simulink model "Gas_Turbine_Model_2017a_non_linear_PID"  (R2021a)
settings: Solver=ode15s  StartTime=0.0  StopTime=90000  FixedStep=0.001  RelTol=1e-3  EnableMultiTasking=on
values from neighbouring files (symbols this model uses):
  Beta_cmp = [1 1.5 2 2.5 3 3.5 4 4.5 5 5.5 6 6.5 ... (39 elements, 39x1)]    [Compressor_Map.mat]
  Eps_turb = [1 1.1 1.2 1.3 1.4 1.5 1.6 1.7 1.8 1.9 2 2.1 ... (191 elements, 1x191)]    [Turbine_Map.mat]
  Eta_cmp = [0.3 0.3 0.3 0.3 0.3 0.3 0.3 0.3 0.3 0.3 0.3 0.3 ... (585 elements, 15x39)]    [Compressor_Map.mat]
  Eta_turb = [0.586812592498 0.603057586725 0.61630240991 0.627098016156 0.635894182286 0.643058088048 0.648889484257 0.653633075447 0.657488628582 0.660619225395 0.663157999268 0.665213634952 ... (191 elements, 1x191)]    [Turbine_Map.mat]
  Mf_cmp = [0.246355651063 0.246355651063 0.246355651063 0.545009157509 1.57043960559 2.28211167924 2.75423550256 3.06528661824 3.27199659823 3.41123925415 3.50631480113 3.5719685441 ... (585 elements, 15x39)]    [Compressor_Map.mat]
  Mf_turb = [1.2124442703 1.39720469175 1.56286841441 1.71140925877 1.84459703271 1.96401861808 2.07109687783 2.16710760884 2.25319474261 2.3303839747 2.39959498557 2.4616523982 ... (191 elements, 1x191)]    [Turbine_Map.mat]
  N_cmp = [30000 35000 40000 45000 50000 55000 60000 65000 70000 75000 80000 85000 ... (15 elements, 1x15)]    [Compressor_Map.mat]
  pow_data = [49.5930192012 49.5930192012 47.1446947685 44.6063090759 42.0564349089 41.1061528351 40.7107031585 40.3152534819 41.8635649412 43.5549903366 45.246415732 45.7100796532 ... (145 elements, 1x145)]    [Pow_demand.mat]
  time_data = [0 600 1200 1800 2400 3000 3600 4200 4800 5400 6000 6600 ... (145 elements, 1x145)]    [Pow_demand.mat]
undefined symbols (not defined in the file or in its folder): cp, cp_m, cv, J, lambda, mf, pamb, Q_LHV, R, sigbuilder_block, Tamb, V
libraries: pid_lib x1
settings Model: Creator=Xinmin Zhang  LastModifiedBy=sandeepsulake
settings SolverCC: ZeroCrossAlgorithm=Adaptive  AlgebraicLoopSolver=TrustRegion
settings DataIOCC: LimitDataPoints=on  SaveFormat=Array  SignalLoggingSaveFormat=ModelDataLogs  ReturnWorkspaceOutputs=off
settings OptimizationCC: ExpressionDepthLimit=2147483647  LifeSpan=inf
settings DebuggingCC: AlgebraicLoopMsg=error  UnderspecifiedInitializationDetection=Classic  MergeDetectMultiDrivingBlocksExec=none  FcnCallInpInsideContextMsg=warning  StateNameClashWarn=warning  SFUnexpectedBacktrackingDiag=warning  SFNoUnconditionalDefaultTransitionDiag=warning  SFExecutionAtInitializationDiag=none  SFMachineParentedDataDiag=warning  ArithmeticOperatorsInVariantConditions=warning
settings HardwareCC: ProdBitPerPointer=32  ProdBitPerSizeT=32  ProdBitPerPtrDiffT=32  ProdLargestAtomicFloat=None  ProdIntDivRoundTo=Undefined  ProdEndianess=Unspecified  ProdWordSize=32  ProdHWDeviceType=32-bit Generic
settings ModelReferenceCC: PropagateSignalLabelsOutOfModel=off
settings SFSimCC: SimUseLocalCustomCode=off  CustomCodeUndefinedFunction=UseInterfaceOnly
settings RTWCC: RTWUseLocalCustomCode=off
settings CodeAppCC: StateflowObjectComments=on
settings GRTTargetCC: TargetLangStandard=C89/C90 (ANSI)  CombineOutputUpdateFcns=off  GRTInterface=on
settings ConfigComp: CovMetricSettings=dw  CovSaveCumulativeToWorkspaceVar=on  CovSaveSingleToWorkspaceVar=on  CovExternalEMLEnable=off

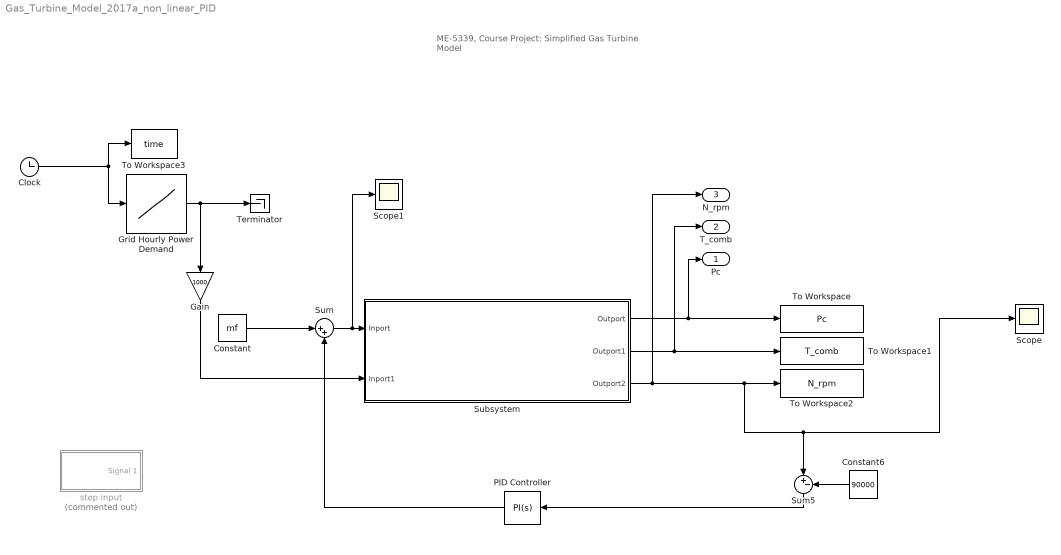
== system Gas_Turbine_Model_2017a_non_linear_PID ==
  note: ME-5339, Course Project:
      | Simplified Gas Turbine Model
  Clock : Clock
  Constant : Constant  Value=mf
  Constant6 : Constant  Value=90000
  Gain : Gain  Gain=1000
  Grid Hourly Power Demand : Lookup_n-D  NumberOfTableDimensions=1  BreakpointsForDimension1=time_data  Table=pow_data  RndMeth=Simplest  InputSameDT=on
  PID Controller : pid_lib/PID Controller  Controller=PI  Form=Parallel  TimeDomain=Continuous-time  UseExternalTs=off  SampleTime=-1  IntegratorMethod=Forward Euler  FilterMethod=Forward Euler  ControllerParametersSource=internal  P=-6.19982666191308e-06  I=-7.95045258926056e-07  D=0  UseFilter=on  N=100  TunerSelectOption=Transfer Function Based (PID Tuner App)  InitialConditionSource=internal  InitialConditionForIntegrator=0  InitialConditionForFilter=0  DifferentiatorICPrevScaledInput=0  ExternalReset=none  TrackingMode=off  Kt=1  LimitOutput=off  SatLimitsSource=internal  UpperSaturationLimit=inf  LowerSaturationLimit=0  LinearizeAsGain=on  AntiWindupMode=none  Kb=1  POutMin=[]  POutMax=[]  IOutMin=[]  IOutMax=[]  DOutMin=[]  DOutMax=[]  NOutMin=[]  NOutMax=[]  SumOutMin=[]  SumOutMax=[]  SaturationOutMin=[]  SaturationOutMax=[]  PParamMin=[]  PParamMax=[]  IParamMin=[]  IParamMax=[]  DParamMin=[]  DParamMax=[]  NParamMin=[]  NParamMax=[]  KbParamMin=[]  KbParamMax=[]  KtParamMin=[]  KtParamMax=[]  KbOutMin=[]  KbOutMax=[]  KtOutMin=[]  KtOutMax=[]  IntegratorOutMin=[]  IntegratorOutMax=[]  FilterOutMin=[]  FilterOutMax=[]  SumI1OutMin=[]  SumI1OutMax=[]  SumI2OutMin=[]  SumI2OutMax=[]  SumI3OutMin=[]  SumI3OutMax=[]  SumI4OutMin=[]  SumI4OutMax=[]  SumDOutMin=[]  SumDOutMax=[]  DifferentiatorOutMin=[]  DifferentiatorOutMax=[]  FilterDiffOutCoefMin=[]  FilterDiffOutCoefMax=[]  ReciprocalOutMin=[]  ReciprocalOutMax=[]  SumDenOutMin=[]  SumDenOutMax=[]  SumNumOutMin=[]  SumNumOutMax=[]  DivideOutMin=[]  DivideOutMax=[]  UdiffTsProdOutMin=[]  UdiffTsProdOutMax=[]  NTsProdOutMin=[]  NTsProdOutMax=[]  UintegralTsProdOutMin=[]  UintegralTsProdOutMax=[]  UngainTsProdOutMin=[]  UngainTsProdOutMax=[]  IntegratorContinuousStateAttributes=''  IntegratorStateMustResolveToSignalObject=off  IntegratorRTWStateStorageClass=Auto  FilterContinuousStateAttributes=''  FilterStateMustResolveToSignalObject=off  FilterRTWStateStorageClass=Auto  ParallelPVariant=InternalParameters  IdealPVariant=Disabled  IVariant=InternalParameters  DVariant=Disabled  IntegratorVariant=Continuous  SatVariant=Disabled  AWVariant=Passthrough  PCopyVariant=Disabled  TRVariant=Disabled  FdbkBlocksVariant=Forward  IdealPFdbkVariant=Disabled  SatFdbkVariant=Disabled  DerivativeFilterVariant=Disabled  NVariant=Disabled  NCopyVariant=Disabled_SignalSpec  FilterICVariant=Disabled  IntegratorICVariant=InternalICs  ExternalResetVariant=Disabled  TRSumVariant=Passthrough  SumFdbkVariant=Disabled  SumVariant=Sum_PI  TsampFilterVariant=InternalTs  TsampNgainVariant=Passthrough  TsampIntegralVariant=Passthrough  ExternalSaturationOutDataTypeStr=Inherit: Same as second input
  Scope : Scope
  Scope1 : Scope
  Subsystem : Subsystem
  Sum : Sum  Inputs=|++
  Sum5 : Sum  Inputs=|+-
  Terminator : Terminator
  To Workspace : ToWorkspace  VariableName=Pc  SampleTime=-1
  To Workspace1 : ToWorkspace  VariableName=T_comb  SampleTime=-1
  To Workspace2 : ToWorkspace  VariableName=N_rpm  SampleTime=-1
  To Workspace3 : ToWorkspace  VariableName=time  SampleTime=-1
  step input : Subsystem  Tag=STV Subsys  Commented=on  LoadFcn=sigbuilder_block('load');  StartFcn=sigbuilder_block('start');  StopFcn=sigbuilder_block('stop');  ClipboardFcn=sigbuilder_block('clipboard');  mask(Sigbuilder block){tuvar=[0:10]}
      mask help: Simulink:masks:SigbuilderBlock_MD
      mask init:
      | if ~strcmp(get_param(bdroot(gcbh),'SimulationStatus'),'stopped') tuvar = sigbuilder_block('maskInit'); end
      settings: CopyFcn=sigbuilder_block('copy');  DeleteFcn=sigbuilder_block('delete');  ModelCloseFcn=sigbuilder_block('modelClose');  PreSaveFcn=sigbuilder_block('preSave');  PauseFcn=sigbuilder_block('pause');  ContinueFcn=sigbuilder_block('continue');  NameChangeFcn=sigbuilder_block('namechange');  OpenFcn=sigbuilder_block('open',[437.6 199.2 550.4 400 ]);  CloseFcn=sigbuilder_block('close');
      mask Display: plot(0, 0, 100, 100,[2, 2, 32, 32, 2], [68, 8, 8, 68, 68],[32, 2], [38, 38], [32, 19, 2],[53, 60, 44], [32, 17, 17, 2],[16, 16, 31, 31]);txt = getActiveGroup(gcbh);text(2, 100, txt,'verticalAlignment', 'top');
  Pc : Outport
  T_comb : Outport  Port=2
  N_rpm : Outport  Port=3
  wires:
  Clock/1 -> To Workspace3/1, Grid Hourly Power Demand/1
  Grid Hourly Power Demand/1 -> Terminator/1, Gain/1
  Subsystem/1(Outport) -> Pc/1, To Workspace/1
  Subsystem/2(Outport1) -> T_comb/1, To Workspace1/1
  Constant/1 -> Sum/1
  Sum5/1 -> PID Controller/1
  Constant6/1 -> Sum5/2
  Subsystem/3(Outport2) -> Scope/1, Sum5/1, To Workspace2/1, N_rpm/1
  PID Controller/1 -> Sum/2
  Sum/1 -> Scope1/1, Subsystem/1(Inport)
  Gain/1 -> Subsystem/2(Inport1)

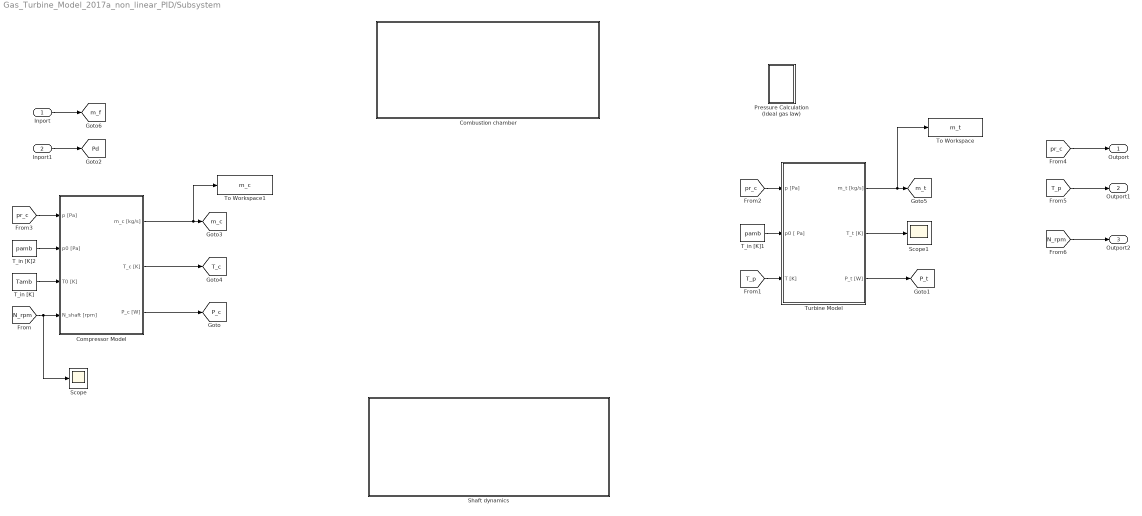
== system Gas_Turbine_Model_2017a_non_linear_PID/Subsystem ==
  Inport : Inport
  Inport1 : Inport  Port=2
  Combustion chamber : Subsystem
  Compressor Model : Subsystem
      mask help: Model of centrifugal compressor
  Pressure Calculation (Ideal gas law) : Subsystem
  Scope : Scope
  Scope1 : Scope
  Shaft dynamics : Subsystem
  T_in [K] : Constant  Value=Tamb
  T_in [K]1 : Constant  Value=pamb
  T_in [K]2 : Constant  Value=pamb
  To Workspace : ToWorkspace  VariableName=m_t  SampleTime=-1
  To Workspace1 : ToWorkspace  VariableName=m_c  SampleTime=-1
  Turbine Model : Subsystem
      mask help: Model of radial inflow turbine
  Outport : Outport
  Outport1 : Outport  Port=2
  Outport2 : Outport  Port=3
  tag scope: P_c=global, P_t=global, Pd=global, T_c=global, m_c=global, m_f=global, m_t=global
  wires:
  Turbine Model/2(T_t [K]) -> Scope1/1
  Compressor Model/3(P_c [W]) -> [P_c]
  [T_p] -> Turbine Model/3(T [K])
  T_in [K]/1 -> Compressor Model/3(T0 [K])
  T_in [K]1/1 -> Turbine Model/2(p0 [ Pa])
  Turbine Model/1(m_t [kg/s]) -> To Workspace/1, [m_t]
  [pr_c] -> Compressor Model/1(p [Pa])
  Compressor Model/2(T_c [K]) -> [T_c]
  T_in [K]2/1 -> Compressor Model/2(p0 [Pa])
  Turbine Model/3(P_t [W]) -> [P_t]
  Compressor Model/1(m_c [kg/s]) -> To Workspace1/1, [m_c]
  [pr_c] -> Turbine Model/1(p [Pa])
  [N_rpm] -> Scope/1, Compressor Model/4(N_shaft [rpm])
  [pr_c] -> Outport/1
  [T_p] -> Outport1/1
  [N_rpm] -> Outport2/1
  Inport/1 -> [m_f]
  Inport1/1 -> [Pd]

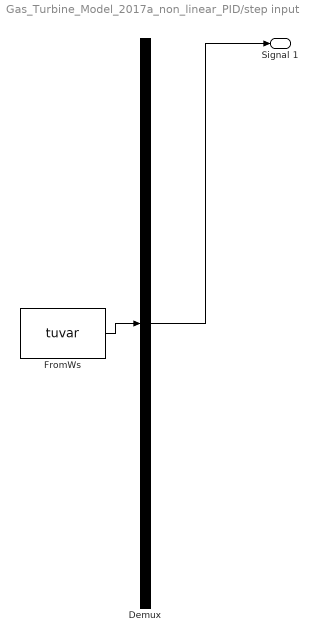
== system Gas_Turbine_Model_2017a_non_linear_PID/step input ==
  Demux : Demux  Tag=STV Demux  Outputs=1
      settings: DisplayOption=none
  FromWs : FromWorkspace  Tag=STV FromWs  VariableName=tuvar
      SigBuilderData=|
      | common.afterFinalStr = 'Extrapolate'
      | common.sampleTime = 0
      | dataSet.timeRange = [0 500]
      | dataSet.name = 'Group 1'
      | sbobj.Groups.Name = 'Group 1'
      | sbobj.Groups.Signals.Name = 'Signal 1'
      | sbobj.Groups.Signals.XData = [0 200 200 300 300 500]
      | sbobj.Groups.Signals.YData = [200000 200000 250000 250000 200000 200000]
      | sbobj.Groups.TimeRange = [0 500]
  Signal 1 : Outport  Tag=STV Outport
  wires:
  FromWs/1 -> Demux/1
  Demux/1 -> Signal 1/1

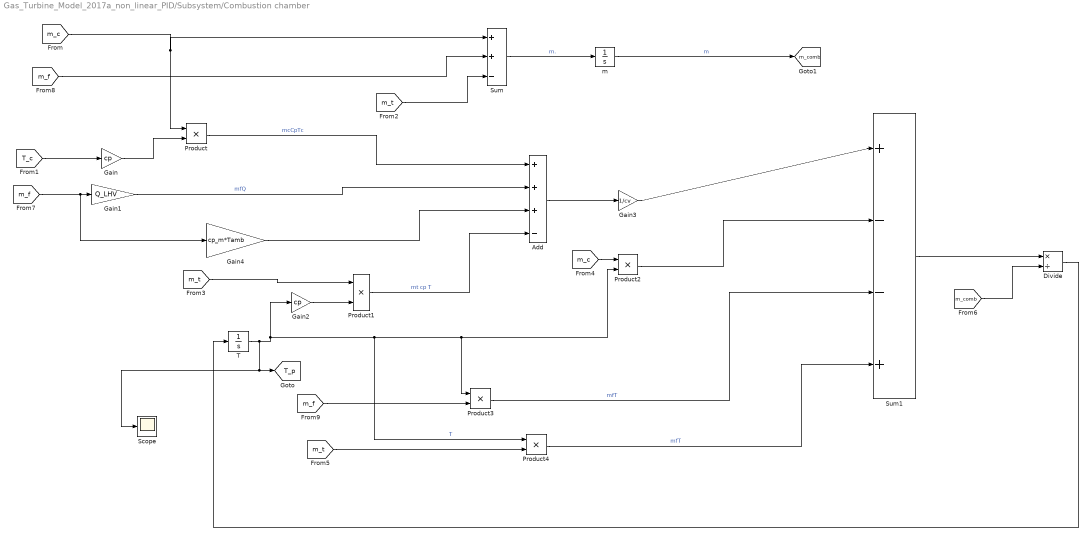
== system Gas_Turbine_Model_2017a_non_linear_PID/Subsystem/Combustion chamber ==
  Add : Sum  Inputs=+++-
  Divide : Product  Inputs=*/
  Gain : Gain  Gain=cp
  Gain1 : Gain  Gain=Q_LHV
  Gain2 : Gain  Gain=cp
  Gain3 : Gain  Gain=1/cv
  Gain4 : Gain  Gain=cp_m*Tamb
  Product{,1..4} (5 alike) : Product
  Scope : Scope
  Sum : Sum  Inputs=|++-
  Sum1 : Sum  Inputs=|+--+
  T : Integrator  InitialCondition=1402.00895175218
  m : Integrator  InitialCondition=6.1482
  tag scope: T_p=global, m_comb=global
  wires:
  m/1 -> [m_comb]  "m"
  [m_f] -> Gain1/1, Gain4/1
  Gain/1 -> Product/2
  Product/1 -> Add/1  "mcCpTc"
  [m_f] -> Sum/2
  Gain1/1 -> Add/2  "mfQ"
  [T_c] -> Gain/1
  Sum/1 -> m/1  "m."
  [m_c] -> Sum/1, Product/1
  [m_t] -> Sum/3
  [m_t] -> Product1/1
  T/1 -> Scope/1, [T_p], Product4/1, Product3/1, Product2/2, Gain2/1  "T"
  Gain2/1 -> Product1/2
  Product1/1 -> Add/4  "mt cp T"
  Add/1 -> Gain3/1
  Gain3/1 -> Sum1/1
  [m_c] -> Product2/1
  Product2/1 -> Sum1/2
  [m_f] -> Product3/2
  Product3/1 -> Sum1/3  "mfT"
  [m_t] -> Product4/2
  Product4/1 -> Sum1/4  "mfT"
  Sum1/1 -> Divide/1
  [m_comb] -> Divide/2
  Divide/1 -> T/1
  Gain4/1 -> Add/3

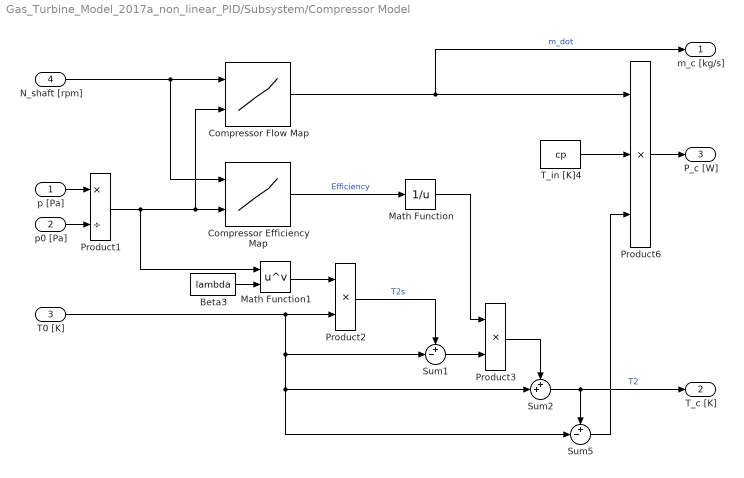
== system Gas_Turbine_Model_2017a_non_linear_PID/Subsystem/Compressor Model ==
  p [Pa] : Inport
  p0 [Pa] : Inport  Port=2
  T0 [K] : Inport  Port=3
  N_shaft [rpm] : Inport  Port=4
  Beta3 : Constant  Value=lambda
  Compressor Efficiency Map : Lookup_n-D  BreakpointsForDimension1=N_cmp  BreakpointsForDimension2=Beta_cmp  Table=Eta_cmp  RndMeth=Simplest  InputSameDT=on
      settings: InputPortMap=u0,u1
  Compressor Flow Map : Lookup_n-D  BreakpointsForDimension1=N_cmp  BreakpointsForDimension2=Beta_cmp  Table=Mf_cmp  RndMeth=Simplest  InputSameDT=on
      settings: InputPortMap=u0,u1
  Math Function : Math  Operator=reciprocal  SignedPower=on  SaturateOnIntegerOverflow=on
  Math Function1 : Math  Operator=pow  SignedPower=on  SaturateOnIntegerOverflow=on
  Product1 : Product  Inputs=*/  RndMeth=Zero
  Product2 : Product  RndMeth=Zero
  Product3 : Product  RndMeth=Zero
  Product6 : Product  Inputs=3  RndMeth=Zero
  Sum1 : Sum  Inputs=+-|
  Sum2 : Sum  Inputs=++|
  Sum5 : Sum  Inputs=+-|
  T_in [K]4 : Constant  Value=cp
  m_c [kg/s] : Outport
  T_c [K] : Outport  Port=2
  P_c [W] : Outport  Port=3
  wires:
  N_shaft [rpm]/1 -> Compressor Efficiency Map/1, Compressor Flow Map/1
  Product1/1 -> Compressor Efficiency Map/2, Compressor Flow Map/2, Math Function1/1
  Compressor Efficiency Map/1 -> Math Function/1  "Efficiency"
  Beta3/1 -> Math Function1/2
  Math Function1/1 -> Product2/1
  Product2/1 -> Sum1/1  "T2s"
  T0 [K]/1 -> Sum1/2, Sum2/2, Sum5/2, Product2/2
  Sum1/1 -> Product3/2
  Math Function/1 -> Product3/1
  Product3/1 -> Sum2/1
  Compressor Flow Map/1 -> m_c [kg/s]/1, Product6/1  "m_dot"
  p [Pa]/1 -> Product1/1
  p0 [Pa]/1 -> Product1/2
  Sum2/1 -> T_c [K]/1, Sum5/1  "T2"
  Product6/1 -> P_c [W]/1
  T_in [K]4/1 -> Product6/2
  Sum5/1 -> Product6/3

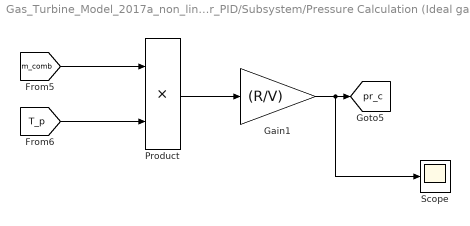
== system Gas_Turbine_Model_2017a_non_linear_PID/Subsystem/Pressure Calculation (Ideal gas law) ==
  Gain1 : Gain  Gain=(R/V)
  Product : Product
  Scope : Scope
  tag scope: pr_c=global
  wires:
  Gain1/1 -> Scope/1, [pr_c]
  [T_p] -> Product/2
  Product/1 -> Gain1/1
  [m_comb] -> Product/1

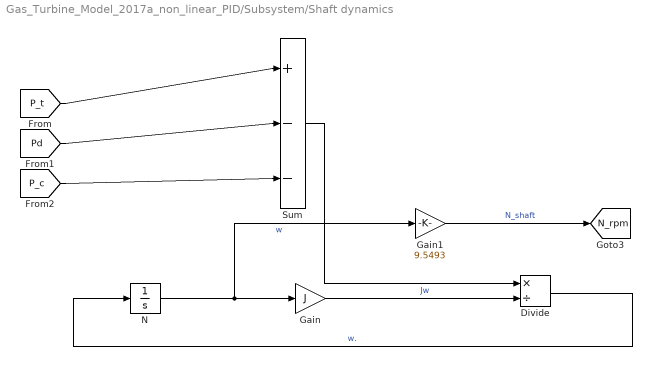
== system Gas_Turbine_Model_2017a_non_linear_PID/Subsystem/Shaft dynamics ==
  Divide : Product  Inputs=*/
  Gain : Gain  Gain=J
  Gain1 : Gain  Gain=9.5493
  N : Integrator  InitialCondition=90723.6250484200*0.104719
  Sum : Sum  Inputs=|+--
  tag scope: N_rpm=global
  wires:
  Divide/1 -> N/1  "w."
  [P_t] -> Sum/1
  [Pd] -> Sum/2
  Gain1/1 -> [N_rpm]  "N_shaft"
  N/1 -> Gain/1, Gain1/1  "w"
  Sum/1 -> Divide/1
  Gain/1 -> Divide/2  "Jw"
  [P_c] -> Sum/3

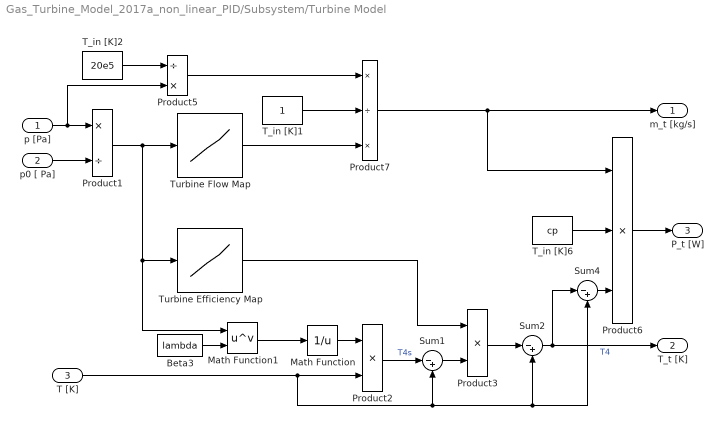
== system Gas_Turbine_Model_2017a_non_linear_PID/Subsystem/Turbine Model ==
  p [Pa] : Inport
  p0 [ Pa] : Inport  Port=2
  T [K] : Inport  Port=3
  Beta3 : Constant  Value=lambda
  Math Function : Math  Operator=reciprocal  SignedPower=on  SaturateOnIntegerOverflow=on
  Math Function1 : Math  Operator=pow  SignedPower=on  SaturateOnIntegerOverflow=on
  Product1 : Product  Inputs=*/  RndMeth=Zero
  Product2 : Product  RndMeth=Zero
  Product3 : Product  RndMeth=Zero
  Product5 : Product  Inputs=/*  RndMeth=Zero
  Product6 : Product  Inputs=3  RndMeth=Zero
  Product7 : Product  Inputs=*/*  RndMeth=Zero
  Sum1 : Sum  Inputs=|-+
  Sum2 : Sum  Inputs=|-+
  Sum4 : Sum  Inputs=|-+
  T_in [K]1 : Constant
  T_in [K]2 : Constant  Value=20e5
  T_in [K]6 : Constant  Value=cp
  Turbine Efficiency Map : Lookup_n-D  NumberOfTableDimensions=1  BreakpointsForDimension1=Eps_turb  Table=Eta_turb  RndMeth=Simplest  InputSameDT=on
  Turbine Flow Map : Lookup_n-D  NumberOfTableDimensions=1  BreakpointsForDimension1=Eps_turb  Table=Mf_turb  RndMeth=Simplest  InputSameDT=on
  m_t [kg/s] : Outport
  T_t [K] : Outport  Port=2
  P_t [W] : Outport  Port=3
  wires:
  Beta3/1 -> Math Function1/2
  Math Function1/1 -> Math Function/1
  T [K]/1 -> Sum4/2, Sum2/2, Sum1/2, Product2/2
  Math Function/1 -> Product2/1
  Product2/1 -> Sum1/1  "T4s"
  Sum1/1 -> Product3/2
  Product3/1 -> Sum2/1
  Sum2/1 -> Sum4/1, T_t [K]/1  "T4"
  T_in [K]6/1 -> Product6/2
  Sum4/1 -> Product6/3
  Turbine Efficiency Map/1 -> Product3/1
  Product6/1 -> P_t [W]/1
  Product1/1 -> Turbine Flow Map/1, Turbine Efficiency Map/1, Math Function1/1
  Turbine Flow Map/1 -> Product7/3
  T_in [K]2/1 -> Product5/1
  Product5/1 -> Product7/1
  T_in [K]1/1 -> Product7/2
  Product7/1 -> m_t [kg/s]/1, Product6/1
  p [Pa]/1 -> Product1/1, Product5/2
  p0 [ Pa]/1 -> Product1/2
